simulink model "data_inspector_full"  (R2024a)
settings: Solver=ode45  StartTime=0.0  StopTime=Sim.time  MaxStep=0.00001  RelTol=1e-12  AbsTol=1e-12
settings Model: Creator=heath  LastModifiedBy=heath

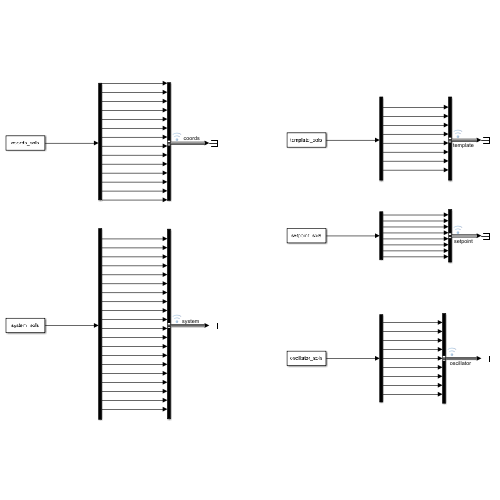
[thumbnail: Simulink's stored preview of the top-level diagram]
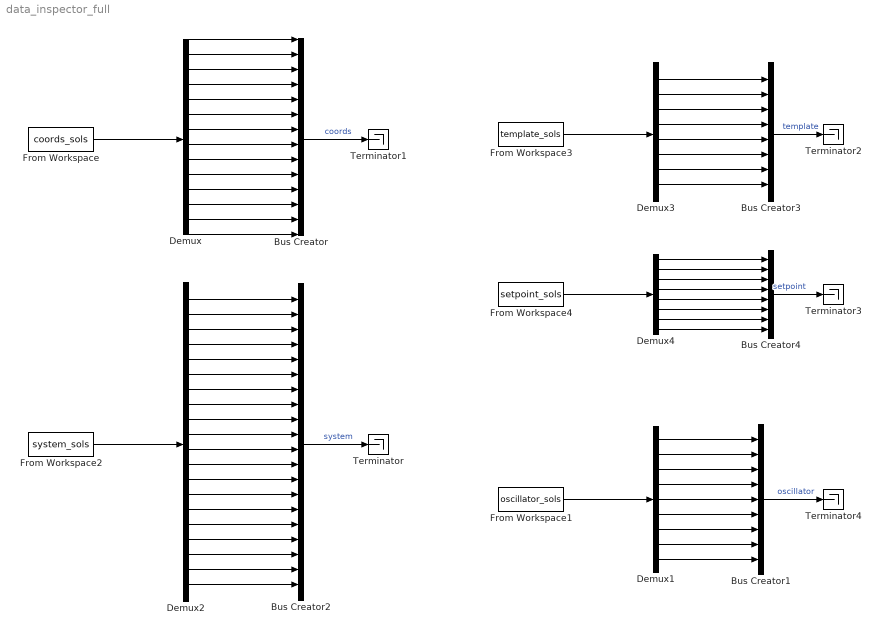
== system data_inspector_full ==
  Bus Creator : BusCreator  Inputs=14  OutDataTypeStr=Bus: Coordinate
      settings: InheritFromInputs=off
  Bus Creator1 : BusCreator  Inputs=9  OutDataTypeStr=Bus: Oscillator
      settings: InheritFromInputs=off
  Bus Creator2 : BusCreator  Inputs=20  OutDataTypeStr=Bus: System
      settings: InheritFromInputs=off
  Bus Creator3 : BusCreator  Inputs=8  OutDataTypeStr=Bus: Template
      settings: InheritFromInputs=off
  Bus Creator4 : BusCreator  Inputs=8  OutDataTypeStr=Bus: Setpoint
      settings: InheritFromInputs=off
  Demux : Demux  Outputs=14
  Demux1 : Demux  Outputs=9
  Demux2 : Demux  Outputs=20
  Demux3 : Demux  Outputs=8
  Demux4 : Demux  Outputs=8
  From Workspace : FromWorkspace  VariableName=coords_sols
  From Workspace1 : FromWorkspace  VariableName=oscillator_sols
  From Workspace2 : FromWorkspace  VariableName=system_sols
  From Workspace3 : FromWorkspace  VariableName=template_sols
  From Workspace4 : FromWorkspace  VariableName=setpoint_sols
  Terminator{,1..4} (5 alike) : Terminator
  wires:
  From Workspace2/1 -> Demux2/1
  From Workspace3/1 -> Demux3/1
  Bus Creator/1 -> Terminator1/1  "coords"
  Demux/8 -> Bus Creator/8
  Demux/7 -> Bus Creator/7
  Demux/6 -> Bus Creator/6
  Demux/5 -> Bus Creator/5
  Demux/4 -> Bus Creator/4
  Demux/3 -> Bus Creator/3
  Demux/2 -> Bus Creator/2
  Demux/1 -> Bus Creator/1
  From Workspace/1 -> Demux/1
  Bus Creator2/1 -> Terminator/1  "system"
  Demux3/1 -> Bus Creator3/1
  Demux3/2 -> Bus Creator3/2
  Demux3/3 -> Bus Creator3/3
  Demux3/4 -> Bus Creator3/4
  Bus Creator3/1 -> Terminator2/1  "template"
  From Workspace4/1 -> Demux4/1
  Demux4/2 -> Bus Creator4/2
  Demux4/1 -> Bus Creator4/1
  Demux4/5 -> Bus Creator4/5
  Demux4/3 -> Bus Creator4/3
  Demux4/4 -> Bus Creator4/4
  Bus Creator4/1 -> Terminator3/1  "setpoint"
  Demux2/9 -> Bus Creator2/9
  Demux2/8 -> Bus Creator2/8
  Demux2/7 -> Bus Creator2/7
  Demux2/6 -> Bus Creator2/6
  Demux2/5 -> Bus Creator2/5
  Demux2/4 -> Bus Creator2/4
  Demux2/3 -> Bus Creator2/3
  Demux2/2 -> Bus Creator2/2
  Demux2/1 -> Bus Creator2/1
  Demux2/10 -> Bus Creator2/10
  Demux2/11 -> Bus Creator2/11
  Demux/9 -> Bus Creator/9
  Demux/10 -> Bus Creator/10
  Demux/11 -> Bus Creator/11
  Demux/12 -> Bus Creator/12
  Demux/13 -> Bus Creator/13
  Demux/14 -> Bus Creator/14
  Demux2/12 -> Bus Creator2/12
  Demux2/13 -> Bus Creator2/13
  Demux2/14 -> Bus Creator2/14
  Demux2/15 -> Bus Creator2/15
  Demux2/16 -> Bus Creator2/16
  Demux2/17 -> Bus Creator2/17
  Demux2/18 -> Bus Creator2/18
  Demux2/19 -> Bus Creator2/19
  Demux2/20 -> Bus Creator2/20
  Demux3/5 -> Bus Creator3/5
  Demux3/6 -> Bus Creator3/6
  Demux3/7 -> Bus Creator3/7
  Demux3/8 -> Bus Creator3/8
  Demux4/6 -> Bus Creator4/6
  Demux4/7 -> Bus Creator4/7
  Demux4/8 -> Bus Creator4/8
  From Workspace1/1 -> Demux1/1
  Demux1/5 -> Bus Creator1/5
  Demux1/4 -> Bus Creator1/4
  Demux1/3 -> Bus Creator1/3
  Demux1/2 -> Bus Creator1/2
  Demux1/1 -> Bus Creator1/1
  Demux1/6 -> Bus Creator1/6
  Demux1/7 -> Bus Creator1/7
  Demux1/9 -> Bus Creator1/9
  Demux1/8 -> Bus Creator1/8
  Bus Creator1/1 -> Terminator4/1  "oscillator"
